simulink model "s01_unicycle"  (R2020a)
settings: Solver=VariableStepAuto  StartTime=0.0  StopTime=20  FixedStep=0.001
InitFcn:
  | clc, close all
  | 
  | run('./s00_config.m')
  | 
  | load('./parameters/ut_obj')
  | load('./parameters/yt_obj')
  | load('./parameters/Kp')
  | load('./parameters/Kr')
  | load('./parameters/Mp')
  | load('./parameters/Mr')
  | 
  | iterSeed = randi(500);
model workspace (MAT data in the model file):
  M = sym
  M.s = 'symobj::fromString("eJytkMGKwjAQhqdWxRW8KYue8gw+wS548ewDlJTMriNJCp262ptP4UP5VCZtwTTiYcGBjxkmP/NnJgWAAcDl6vIwTUYufa2gjdTV8652GvjwcM2SmX5t0+69rz0npFKJP1mSzDUKKw2yODIqQVZwbYr8sDkaU28V2op+CEsIPQfRzKFnX2gVaV79sdGzLqqoP/ZwpTTljd8UHjHzMFa72nxrkozc7rYMPG6B/m0HW3he3uR/R4m9m4UzsgrPT74TT+aMpeXMvX0GM9Jgz0R0Oep30dd2Q5I7SlFCoD==", 2)'
  M.Digits = 32
  M_nonlin = sym
  M_nonlin.s = 'symobj::fromString("eJytkMGKwjAQhqdWxRW8KYue8gw+wS548ewDlJTMriNJCp262ptP4UP5VCZtwTTiYcGBjxkmP/NnJgWAAcDl6vIwTUYufa2gjdTV8652GvjwcM2SmX5t0+69rz0npFKJP1mSzDUKKw2yODIqQVZwbYr8sDkaU28V2op+CEsIPQfRzKFnX2gVaV79sdGzLqqoP/ZwpTTljd8UHjHzMFa72nxrkozc7rYMPG6B/m0HW3he3uR/R4m9m4UzsgrPT74TT+aMpeXMvX0GM9Jgz0R0Oep30dd2Q5I7SlFCoD==", 2)'
  M_nonlin.Digits = 32
  M_tmp = sym
  M_tmp.s = 'symobj::fromString("eJytUMGKwkAMTa0uruBNcfU037BfsIIXz35AmTJxjcxMoamrvfkVfpRf5UxbcBzxIGzg8ULyyEuSAkAP4Hxx3E+TgaOfBbSRunzS5U4Dnx5cs2SmX9uUH/rfHkekUok/WZLMNQorDbI4MCpBVnBtiny/OhhTrxXairaEJYSevWhm32NXaBVpXu3Y6FkXVVT/8OBKacobvxHcY+zBWG1qs9QkGbm9bR54XAP9vz1s6vHyJ+89JfZuDs7IKjw9+Q49MmcsLWeuNwtmpMGdieg4qnfxqP3q+AZKWUKh", 2)'
  M_tmp.Digits = 32
  RHS = sym
  RHS.s = 'symobj::fromString("eJytUMGKwkAMTa2KK3hTFj3NN/gFu+DFsx9Qpkx2jcxMoamrvfkVfpRf5UxbcDriYcHAIyF55CUvBYABwOXq8jBNRi59raCN1NXzrnYc+PDgmiUz/dqm3ZuvPU5IpRJ/siSZaxRWGmRxZFSCrODaFPlhczSm3iq0Ff0QlhBqDqKdQ499oVXEeXVjw2ddVFF/7MGV0pQ3elN4xMyDsdrV5luTZOT2t2WgcQv4bzNs4fHSk/+ZEms3D2dkFZ6fdCcemROWljM3+wx2pMGfiehy1O+iz+3cSu5KYUKi", 2)'
  RHS.Digits = 32
  RHS_nonlin = sym
  RHS_nonlin.s = 'symobj::fromString("eJytUMGKwkAMTa2KK3hTFj3NN/gFu+DFsx9Qpkx2jcxMoamrvfkVfpRf5UxbcDriYcHAIyF55CUvBYABwOXq8jBNRi59raCN1NXzrnYc+PDgmiUz/dqm3ZuvPU5IpRJ/siSZaxRWGmRxZFSCrODaFPlhczSm3iq0Ff0QlhBqDqKdQ499oVXEeXVjw2ddVFF/7MGV0pQ3elN4xMyDsdrV5luTZOT2t2WgcQv4bzNs4fHSk/+ZEms3D2dkFZ6fdCcemROWljM3+wx2pMGfiehy1O+iz+3cSu5KYUKi", 2)'
  RHS_nonlin.Digits = 32
  RHS_tmp = sym
  RHS_tmp.s = 'symobj::fromString("eJytUMGKwkAMTa2KK3hTFj3NN/gFu+DFsx9Qpkx2jcxMoamrvfkVfpRf5UxbcDriYcHAIyF55CUvBYABwOXq8jBNRi59raCN1NXzrnYc+PDgmiUz/dqm3ZuvPU5IpRJ/siSZaxRWGmRxZFSCrODaFPlhczSm3iq0Ff0QlhBqDqKdQ499oVXEeXVjw2ddVFF/7MGV0pQ3elN4xMyDsdrV5luTZOT2t2WgcQv4bzNs4fHSk/+ZEms3D2dkFZ6fdCcemROWljM3+wx2pMGfiehy1O+iz+0OSe5KaUKj", 2)'
  RHS_tmp.Digits = 32
  Tp = sym
  Tp.s = 'symobj::fromString("eJytUMGKwkAMTa0uruBNkdXLfMN+wQpePPsBZcrENTIzhaau9uZX+FF+lTNtwXHEg7CBxwvJIy9JCgA9gPPFcT9NBo5+5tBG6vJJlzsNfHpwzZKZfm1Tfuh/exyRSiX+ZEky1yisNMjiwKgEWcG1KfL96mBMvVZoK9oSlhB69qKZfY9doVWkebVjo2ddVFH9w4MrpSlv/EZwj7EHY7WpzVKTZOT2tq/A4xro/+1hU4+XP3nvKbF3c3BGVuHpyXfokTljaTlzvVkwIw3uTETHUb2LR+2i4xtKcUKk", 2)'
  Tp.Digits = 32
  Tp_var = 0
  Tw = sym
  Tw.s = 'symobj::fromString("eJytUMGKwkAMTa0uruBNkRUP8w37BSt48ewHlCkT18jMFJq62ptf4Uf5Vc60BccRD8IGHi8kj7wkKQD0AM4Xx/00GTj6mUMbqcsnXe408OnBNUtm+rVN+aH/7XFEKpX4kyXJXKOw0iCLA6MSZAXXpsj3q4Mx9VqhrWhLWELo2Ytm9j12hVaR5tWOjZ51UUX1Dw+ulKa88RvBPcYejNWmNktNkpHb274Cj2ug/7eHTT1e/uS9p8TezcEZWYWnJ9+hR+aMpeXM9WbBjDS4MxEdR/UuHrWLjm9KeUKl", 2)'
  Tw.Digits = 32
  Tw_var = 0
  op_trim3 : handle (value not decoded)
  q1 = sym
  q1.s = 'symobj::fromString("eJytUFGKwkAMTa0uruCfIisIc4Y9wQr++O0BypSJa2RmCk1d7Z+n8FCeypm24Djih7CBxwvJIy9JCgA9gPPFcT9NBo5+5tBG6vJJlzsNfHpwzZKZfm1Tfuh/exyRSiX+ZEky1yisNMjiwKgEWcG1KfL96mBMvVZoK9oSlhB69qKZfY9doVWkebVjo2ddVFH9w4MrpSlv/EZwj7EHY7WpzVKTZOT2tq/A4xro/+1hU4+XP3nvKbF3c3BGVuHpyXfokTljaTlzvVkwIw3uTETHUb2LR+2i4xtKgUKm", 2)'
  q1.Digits = 32
  q1_d = sym
  q1_d.s = 'symobj::fromString("eJytUMGKwkAMTa0uruBNkfUg8w37BSt48ewHlCkT18jMFJq62ptf4Uf5Vc60BccRD8IGHi8kj7wkKQD0AM4Xx/00GTj6mUMbqcsnXe408OnBNUtm+rVN+aH/7XFEKpX4kyXJXKOw0iCLA6MSZAXXpsj3q4Mx9VqhrWhLWELo2Ytm9j12hVaR5tWOjZ51UUX1Dw+ulKa88RvBPcYejNWmNktNkpHb274Cj2ug/7eHTT1e/uS9p8TezcEZWYWnJ9+hR+aMpeXM9WbBjDS4MxEdR/UuHrWLjm9KiUKn", 2)'
  q1_d.Digits = 32
  q2 = sym
  q2.s = 'symobj::fromString("eJytUMGKwkAMTa0uruBNkfXifMN+wQpePPsBZcrENTIzhaau9uZX+FF+lTNtwXHEg7CBxwvJIy9JCgA9gPPFcT9NBo5+5tBG6vJJlzsNfHpwzZKZfm1Tfuh/exyRSiX+ZEky1yisNMjiwKgEWcG1KfL96mBMvVZoK9oSlhB69qKZfY9doVWkebVjo2ddVFH9w4MrpSlv/EZwj7EHY7WpzVKTZOT2tq/A4xro/+1hU4+XP3nvKbF3c3BGVuHpyXfokTljaTlzvVkwIw3uTETHUb2LR+2i4xtKkUKo", 2)'
  q2.Digits = 32
  q2_d = sym
  q2_d.s = 'symobj::fromString("eJytUEGOwjAMdGlBLBK3RQhOeQMvYCUunHlAlSpmMUpSqS679MYr+BO8apNSiZAVByQsjezYI088KQD0AE5nl7M06bu0nMMtUld/drXjwIcHNyyZ6du27Yf5wuMXqVLiR1YkC43CSoMsDoxKkBXcmLLYrw7GNGuFtqYtYQWhZi/amXnsSq0izrM/tnzWZR31Bx5cK01FqzeCe4w9GOtNY740SUa+3TYLNK4B/22GTTyeevKaKbF2e3BOVuHxn+7QI3fC0nLuZtNgRxrcmYguR/0ulpfgMfgDP01DUz==", 2)'
  q2_d.Digits = 32
  q3 = sym
  q3.s = 'symobj::fromString("eJytUEuKAkEMTds6zAjuFBlXNVeYEyi4ce0BmmoqjpGqaui0n955Cg/lqazqbrAscSFM4PFC8shLkgJAD+B8cdxPk4Gj+QzaSF0+7nKngS8Prlky059tyg/9X48jUqnEQZYkc43CSoMs9oxKkBVcmyLfLffG1CuFtqINYQmhZy+a2ffYFlpFmlc7NnrWRRXVPzy4Upryxm8I9xh5MFbr2iw0SUZub/sOPK6B/t8eNvF4+ZP3nhJ7NwdnZBWennw/PTJnLC1nrjcNZqTBnYnoOKp38aj96fgGSqFCqj==", 2)'
  q3.Digits = 32
  q3_d = sym
  q3_d.s = 'symobj::fromString("eJytUEuKAkEMTds6zAjuFBlXxRxhTqDgxrUHaKqpOEaqqqHTfnrnKTyUp7Kqu8GyxIUwgccLySMvSQoAPYDzxXE/TQaO5jNoI3X5uMudBr48uGbJTH+2KT/0fz2OSKUSB1mSzDUKKw2y2DMqQVZwbYp8t9wbU68U2oo2hCWEnr1oZt9jW2gVaV7t2OhZF1VU//DgSmnKG78h3GPkwVita7PQJBm5ve078LgG+n972MTj5U/ee0rs3RyckVV4evL99MicsbScud40mJEGdyai46jexaP2p+MbSqlCqz==", 2)'
  q3_d.Digits = 32
  q4 = sym
  q4.s = 'symobj::fromString("eJytUEuKAkEMTds6zAjuFBlXBXODOYGCG9ceoKmm4hipqoZO++mdp/BQnsqq7gbLEhfCBB4vJI+8JCkA9ADOF8f9NBk4ms+gjdTl4y53Gvjy4JolM/3ZpvzQ//U4IpVKHGRJMtcorDTIYs+oBFnBtSny3XJvTL1SaCvaEJYQevaimX2PbaFVpHm1Y6NnXVRR/cODK6Upb/yGcI+RB2O1rs1Ck2Tk9rbvwOMa6P/tYROPlz957ymxd3NwRlbh6cn30yNzxtJy5nrTYEYa3JmIjqN6F4/an45vSrFCrD==", 2)'
  q4.Digits = 32
  q4_d = sym
  q4_d.s = 'symobj::fromString("eJytUEuKAkEMTds6zAjuFBlXtZgTzAkU3Lj2AE01FcdIVTV02k/vPIWH8lRWdTdYlrgQJvB4IXnkJUkBoAdwvjjup8nA0XwGbaQuH3e508CXB9csmenPNuWH/q/HEalU4iBLkrlGYaVBFntGJcgKrk2R75Z7Y+qVQlvRhrCE0LMXzex7bAutIs2rHRs966KK6h8eXClNeeM3hHuMPBirdW0WmiQjt7d9Bx7XQP9vD5t4vPzJe0+JvZuDM7IKT0++nx6ZM5aWM9ebBjPS4M5EdBzVu3jU/nR8A0q5Qq0=", 2)'
  q4_d.Digits = 32
  q5 = sym
  q5.s = 'symobj::fromString("eJytUEuKAkEMTds6zAjuFBlXtZkLzAkU3Lj2AE01FcdIVTV02k/vPIWH8lRWdTdYlrgQJvB4IXnkJUkBoAdwvjjup8nA0XwGbaQuH3e508CXB9csmenPNuWH/q/HEalU4iBLkrlGYaVBFntGJcgKrk2R75Z7Y+qVQlvRhrCE0LMXzex7bAutIs2rHRs966KK6h8eXClNeeM3hHuMPBirdW0WmiQjt7d9Bx7XQP9vD5t4vPzJe0+JvZuDM7IKT0++nx6ZM5aWM9ebBjPS4M5EdBzVu3jU/nR8A0rBQq4=", 2)'
  q5.Digits = 32
  q5_d = sym
  q5_d.s = 'symobj::fromString("eJytUEuKAkEMTds6zAjuFBlXtZoDzAkU3Lj2AE01FcdIVTV02k/vPIWH8lRWdTdYlrgQJvB4IXnkJUkBoAdwvjjup8nA0XwGbaQuH3e508CXB9csmenPNuWH/q/HEalU4iBLkrlGYaVBFntGJcgKrk2R75Z7Y+qVQlvRhrCE0LMXzex7bAutIs2rHRs966KK6h8eXClNeeM3hHuMPBirdW0WmiQjt7d9Bx7XQP9vD5t4vPzJe0+JvZuDM7IKT0++nx6ZM5aWM9ebBjPS4M5EdBzVu3jU/nR8A0rJQq8=", 2)'
  q5_d.Digits = 32
  z = [0  0  0  0  0  0  0  0  0  0; 0  0  0  0  0  0  0  0  0  0; 0  0  0  0  0  0  0  0  0  0; 0  0  0  0  0  0  0  0  0  0; 0  0  0  0  0  0  0  0  0  0; 0  0  0  0  0  0  0  0  0  0; 0  0  0  0  0  0  0  0  0  0; 0  0  0  0  0  0  0  0  0  0; 0  0  0  0  0  0  0  0  0  0; 0  0  0  0  0  0  0  0  0  0]
values from neighbouring files (symbols this model uses):
  b_disc = 0.01    [s00_config.m]
  Bp = [B_p1 B_p2 B_p3 B_p4]    [s00_config.m]    (also in s00_designLQR.m = double([0; b2; 0; b4]))
  flag_AddPitchBias = 0    [s00_config.m]
  flag_AddRollBias = 0    [s00_config.m]
  flag_UseAccNoise = 1    [s00_config.m]
  flag_useControlDelay = 0    [s00_config.m]
  flag_UseGyroNoise = 1    [s00_config.m]
  flag_UsePitchEst = 1    [s00_config.m]
  flag_UsePivotAcc = 1    [s00_config.m]
  flag_UseRateEst = 1    [s00_config.m]
  flag_UseRollEst = 1    [s00_config.m]
  flag_UseYawEst = 1    [s00_config.m]
  Icx = 0.001746    [s00_config.m]
  Icy = 0.00181    [s00_config.m]
  Icz = 0.001585    [s00_config.m]
  Iwx = 0.000259    [s00_config.m]
  Iwy = 0.000503    [s00_config.m]
  Iwz = 0.000259    [s00_config.m]
  Lc = 0.055    [s00_config.m]
  Lcp = 0.055    [s00_config.m]
  mean_IMUgyro = -0.0065    [s00_config.m]
  pitch_bias = deg2rad(1)    [s00_config.m]
  q1_0 = -deg2rad(36)    [s00_config.m]
  q2_0 = deg2rad(0)    [s00_config.m]
  r = Rw - 0.01    (= 0.043)    [s00_config.m]
  roll_bias = deg2rad(1)    [s00_config.m]
  Rw = 0.053    [s00_config.m]
  stall_torque = 1.6    [s00_config.m]
  Ts = 1/100    (= 0.01)    [s00_config.m]
  variance_IMUacc = 0.0049    [s00_config.m]
  variance_IMUgyro = 6.3956e-04    (= 0.00063956)    [s00_config.m]
  X = (P.')/(P*P.')    [s00_config.m]
  Xp = X(:,1)    [s00_config.m]
undefined symbols (not defined in the file or in its folder): DiscIntNeverNeededParam, sigbuilder_block, Y, Z
libraries: sm_lib x59, aerolibconvert2 x11, nesl_utility x8, eeGeneralControl x2, simulink x1, SignalEditorBlockLib x1
(part 1 of 2)
settings Model: Creator=zjia  LastModifiedBy=Geist
settings DataIOCC: ExternalInput=getinputstruct(op_trim3)  InitialState=getstatestruct(op_trim3)  ReturnWorkspaceOutputs=off
settings DebuggingCC: PregeneratedLibrarySubsystemCodeDiagnostic=none  ArithmeticOperatorsInVariantConditions=warning
settings SFSimCC: SimUseLocalCustomCode=off  CustomCodeUndefinedFunction=UseInterfaceOnly
settings RTWCC: RTWUseLocalCustomCode=off
settings ExplorerConfigSet: InternalSimMechanicsExplorerSettings="<ExplorerConfiguration><canonicalview>default</canonicalview><AnimationSetting><BasePlaybackSpeed>1.0</BasePlaybackSpeed><PlaybackSpeedFactor>1.0</PlaybackSpeedFactor></AnimationSetting><TilePanel><TileInfo><Tiles Columns=\"1\" Count=\"1\" Rows=\"1\"><Column Weight=\"1\"/><Row Weight=\"1\"/><Tile Height=\"1\" Width=\"1\" X=\"0\" Y=\"0\"/></Tiles></TileInfo><SceneInfo><SceneViewer><BGColor><R>0.60000002384185791</R><G>0.60000002384185791</G><B>0.60000002384185791</B></BGColor><Camera><DoPerspective>off</DoPerspective><Position><X>-1.31570593920536782</X><Y>-1.95913294447027075</Y><Z>2.91484294326524562</Z></Position><Center><X>-0.265965718532476025</X><Y>-0.0141378650214136238</Y><Z>0.259288232843852717</Z></Center><Up><X>0.409238570116308875</X><Y>0.651418880522143251</Y><Z>0.638887497786924219</Z></Up><ViewLimDist>1</ViewLimDist><YLim>0.274439838409632098</YLim><XLim>0.321907563939727526</XLim></Camera></SceneViewer></SceneInfo></TilePanel><MechEditorPanel><Cameras/><GfxPanelCameraMap/><VideoCreator><PlaybackSpeedRatio>1.0</PlaybackSpeedRatio><FrameRate>30</FrameRate><VideoFormat>Motion JPEG AVI</VideoFormat><FrameSize>auto</FrameSize></VideoCreator></MechEditorPanel></ExplorerConfiguration>"

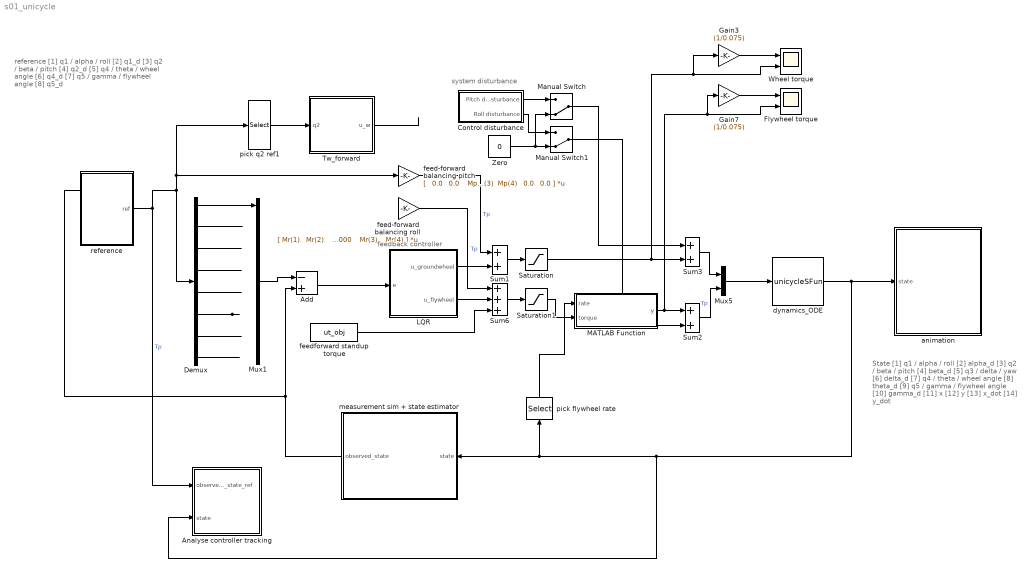
== system s01_unicycle ==
  note: State
      |
      | [1] q1 / alpha / roll
      | [2] alpha_d
      | [3] q2 / beta / pitch
      | [4] beta_d
      | [5] q3 / delta / yaw
      | [6] delta_d
      | [7] q4 / theta / wheel angle
      | [8] theta_d
      | [9] q5 / gamma / flywheel angle
      | [10] gamma_d
      | [11] x
      | [12] y
      | [13] x_dot
      | [14] y_dot
  note: feedback controller
  note: reference
      |
      | [1] q1 / alpha / roll
      | [2] q1_d
      | [3] q2 / beta / pitch
      | [4] q2_d
      | [5] q4 / theta / wheel angle
      | [6] q4_d
      | [7] q5 / gamma / flywheel angle
      | [8] q5_d
  note: system disturbance
  Add : Sum  Inputs=-+
  Analyse controller tracking : Subsystem
  Control disturbance : Subsystem  Tag=STV Subsys  LoadFcn=sigbuilder_block('load');  StartFcn=sigbuilder_block('start');  StopFcn=sigbuilder_block('stop');  ClipboardFcn=sigbuilder_block('clipboard');  mask(Sigbuilder block){tuvar=[0:10]}
      mask help: Simulink:masks:SigbuilderBlock_MD
      mask init:
      | if ~strcmp(get_param(bdroot(gcbh),'SimulationStatus'),'stopped') tuvar = sigbuilder_block('maskInit'); end
      settings: CopyFcn=sigbuilder_block('copy');  DeleteFcn=sigbuilder_block('delete');  ModelCloseFcn=sigbuilder_block('modelClose');  PreSaveFcn=sigbuilder_block('preSave');  PauseFcn=sigbuilder_block('pause');  ContinueFcn=sigbuilder_block('continue');  NameChangeFcn=sigbuilder_block('namechange');  OpenFcn=sigbuilder_block('open',[437.6 199.2 550.4 400 ]);  CloseFcn=sigbuilder_block('close');
      mask Display: plot(0, 0, 100, 100,[2, 2, 32, 32, 2], [68, 8, 8, 68, 68],[32, 2], [38, 38], [32, 19, 2],[53, 60, 44], [32, 17, 17, 2],[16, 16, 31, 31]);txt = getActiveGroup(gcbh);text(2, 100, txt,'verticalAlignment', 'top');
  Demux : Demux  Outputs=8
  Flywheel torque : Scope  NumInputPorts=2
  Gain3 : Gain  Gain=(1/0.075)
  Gain7 : Gain  Gain=(1/0.075)
  LQR : Subsystem
  MATLAB Function : MATLAB Function  TreatAsAtomicUnit=on
  Manual Switch : ManualSwitch  CurrentSetting=0
  Manual Switch1 : ManualSwitch  CurrentSetting=0
  Mux1 : Mux  Inputs=8
  Mux5 : Mux  Inputs=2
  Saturation : Saturate  UpperLimit=stall_torque  LowerLimit=-stall_torque
  Saturation1 : Saturate  UpperLimit=stall_torque  LowerLimit=-stall_torque
  Sum1 : Sum
  Sum2 : Sum
  Sum3 : Sum
  Sum6 : Sum  Inputs=+++
  Tw_forward : MATLAB Function  TreatAsAtomicUnit=on
  Wheel torque : Scope  NumInputPorts=2
  Zero : Constant  Value=0  OutDataTypeStr=Inherit: Inherit via back propagation
  animation : Subsystem
      mask Display: image('C:\Users\geist\Documents\code_projects\uniwheel_model\simulink_3D_unicycle\images\simulation_block_image.PNG'); % Use "Edit Image" on toolstrip to change.
  dynamics_ODE : S-Function  FunctionName=unicycleSFun  SFunctionDeploymentMode=off  EnableBusSupport=off
  feed-forward balancing pitch : Gain  Gain=|  Multiplication=Matrix(K*u) (u vector)
      | [   0.0   0.0    Mp(1)   Mp(2)   Mp(3)  Mp(4)   0.0   0.0
      | ]
  feed-forward balancing roll : Gain  Gain=|  Multiplication=Matrix(K*u) (u vector)
      | [ Mr(1)   Mr(2)    0.0000    0.0000    0.0000    0.0000    Mr(3)    Mr(4)
      | ]
  feedforward standup torque : FromWorkspace  VariableName=ut_obj
  measurement sim + state estimator : Subsystem
  pick flywheel rate : Selector  InputPortWidth=14  IndexOptions=Index vector (dialog)  Indices=[10]  OutputSizes=1
  pick q2 ref1 : Selector  InputPortWidth=8  IndexOptions=Index vector (dialog)  Indices=[3]  OutputSizes=1
  reference : Subsystem
  wires:
  Mux5/1 -> dynamics_ODE/1
  Sum3/1 -> Mux5/1
  measurement sim + state estimator/1(observed_state) -> Add/2
  Sum2/1 -> Mux5/2  "Tp"
  Manual Switch1/1 -> Sum2/2
  MATLAB Function/1(y) -> Sum2/1, Flywheel torque/2, Gain7/1
  Control disturbance/1(Pitch disturbance) -> Manual Switch/1
  Manual Switch/1 -> Sum3/1
  Zero/1 -> Manual Switch1/2, Manual Switch/2
  Control disturbance/2(Roll disturbance) -> Manual Switch1/1
  Gain3/1 -> Wheel torque/1
  Gain7/1 -> Flywheel torque/1
  pick flywheel rate/1 -> MATLAB Function/1(rate)
  feedforward standup torque/1 -> Sum6/3
  Sum6/1 -> Saturation1/1
  Add/1 -> LQR/1(e)
  feed-forward balancing pitch/1 -> Sum1/1  "Tp"
  Sum1/1 -> Saturation/1
  feed-forward balancing roll/1 -> Sum6/1  "Tp"
  dynamics_ODE/1 -> Analyse controller tracking/2(state), pick flywheel rate/1, measurement sim + state estimator/1(state), animation/1(state)
  LQR/1(u_groundwheel) -> Sum1/2
  LQR/2(u_flywheel) -> Sum6/2
  Saturation/1 -> Sum3/2, Gain3/1, Wheel torque/2
  Saturation1/1 -> MATLAB Function/2(torque)
  reference/1(ref) -> feed-forward balancing pitch/1, pick q2 ref1/1, Demux/1, Analyse controller tracking/1(observed_state_ref)  "Tp"
  Demux/3 -> ?
  Demux/6 -> ?
  Mux1/1 -> Add/1
  Demux/2 -> ?
  Demux/1 -> Mux1/1
  Demux/8 -> ?
  Demux/7 -> ?
  Demux/5 -> ?
  Demux/4 -> ?
  Tw_forward/1(u_w) -> ?
  pick q2 ref1/1 -> Tw_forward/1(q2)

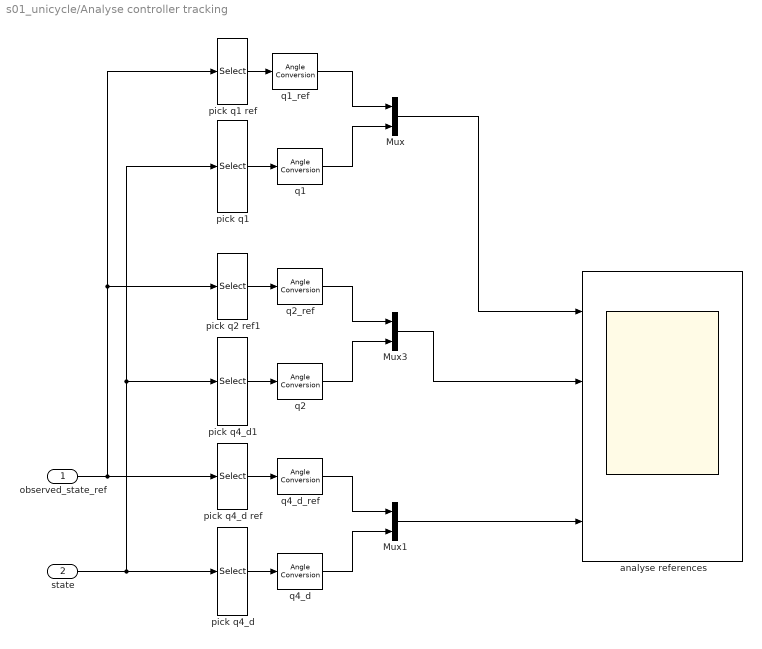
== system s01_unicycle/Analyse controller tracking ==
  observed_state_ref : Inport
  state : Inport  Port=2
  Mux : Mux  Inputs=2
  Mux1 : Mux  Inputs=2
  Mux3 : Mux  Inputs=2
  analyse references : Scope  NumInputPorts=4
  pick q1 : Selector  InputPortWidth=14  IndexOptions=Index vector (dialog)  Indices=[1]  OutputSizes=1
  pick q1 ref : Selector  InputPortWidth=8  IndexOptions=Index vector (dialog)  Indices=[1]  OutputSizes=1
  pick q2 ref1 : Selector  InputPortWidth=8  IndexOptions=Index vector (dialog)  Indices=[3]  OutputSizes=1
  pick q4_d : Selector  InputPortWidth=14  IndexOptions=Index vector (dialog)  Indices=[8]  OutputSizes=1
  pick q4_d ref : Selector  InputPortWidth=8  IndexOptions=Index vector (dialog)  Indices=[6]  OutputSizes=1
  pick q4_d1 : Selector  InputPortWidth=14  IndexOptions=Index vector (dialog)  Indices=[3]  OutputSizes=1
  q1 : aerolibconvert2/Angle Conversion  IU=rad  OU=deg
  q1_ref : aerolibconvert2/Angle Conversion  IU=rad  OU=deg
  q2 : aerolibconvert2/Angle Conversion  IU=rad  OU=deg
  q2_ref : aerolibconvert2/Angle Conversion  IU=rad  OU=deg
  q4_d : aerolibconvert2/Angle Conversion  IU=rad  OU=deg
  q4_d_ref : aerolibconvert2/Angle Conversion  IU=rad  OU=deg
  wires:
  pick q4_d ref/1 -> q4_d_ref/1
  pick q4_d/1 -> q4_d/1
  q1/1 -> Mux/2
  pick q1/1 -> q1/1
  observed_state_ref/1 -> pick q2 ref1/1, pick q1 ref/1, pick q4_d ref/1
  pick q1 ref/1 -> q1_ref/1
  q4_d_ref/1 -> Mux1/1
  q1_ref/1 -> Mux/1
  q4_d/1 -> Mux1/2
  Mux1/1 -> analyse references/4
  Mux/1 -> analyse references/1
  Mux3/1 -> analyse references/2
  q2/1 -> Mux3/2
  q2_ref/1 -> Mux3/1
  state/1 -> pick q4_d1/1, pick q1/1, pick q4_d/1
  pick q4_d1/1 -> q2/1
  pick q2 ref1/1 -> q2_ref/1

== system s01_unicycle/Control disturbance ==
  Demux : Demux  Tag=STV Demux  Outputs=2
      settings: DisplayOption=none
  FromWs : FromWorkspace  Tag=STV FromWs  VariableName=tuvar
      SigBuilderData=|
      | common.afterFinalStr = 'Extrapolate'
      | common.sampleTime = 0
      | dataSet.timeRange = [0 10]
      | dataSet.name = 'Group 1'
      | sbobj.Groups.Name = 'Group 1'
      | sbobj.Groups.Signals(1).Name = 'Pitch disturbance'
      | sbobj.Groups.Signals(1).XData = [0 2.9 3 3.1 3.2 10]
      | sbobj.Groups.Signals(1).YData = [0 0 0.272 0.128 0 0]
      | sbobj.Groups.Signals(2).Name = 'Roll disturbance'
      | sbobj.Groups.Signals(2).XData = [0 2.9 3 3.2 3.3 10]
      | sbobj.Groups.Signals(2).YData = [0 0 0.505 0.185 0 0]
  Pitch disturbance : Outport  Tag=STV Outport
  Roll disturbance : Outport  Tag=STV Outport  Port=2
  wires:
  Demux/1 -> Pitch disturbance/1
  FromWs/1 -> Demux/1
  Demux/2 -> Roll disturbance/1

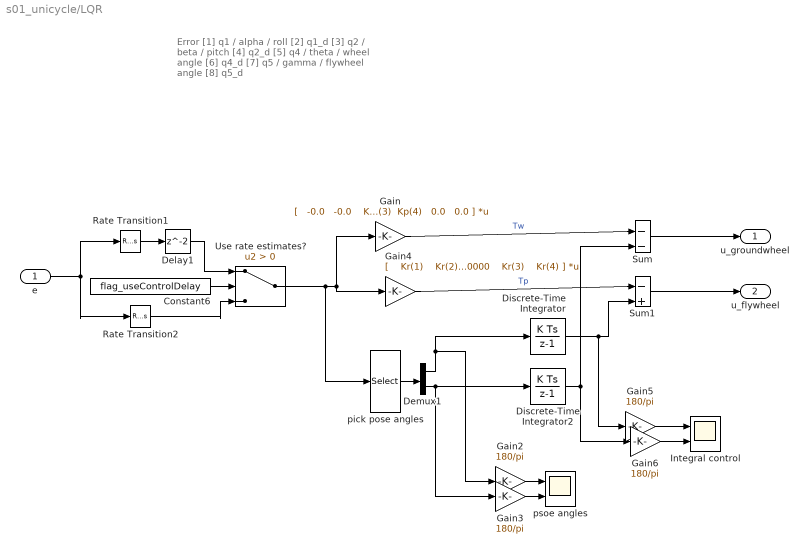
== system s01_unicycle/LQR ==
  note: Error
      |
      | [1] q1 / alpha / roll
      | [2] q1_d
      | [3] q2 / beta / pitch
      | [4] q2_d
      | [5] q4 / theta / wheel angle
      | [6] q4_d
      | [7] q5 / gamma / flywheel angle
      | [8] q5_d
  e : Inport
  Constant6 : Constant  Value=flag_useControlDelay
  Delay1 : Delay  SampleTime=Ts
  Demux1 : Demux  Outputs=2
  Discrete-Time Integrator : DiscreteIntegrator  gainval=gain_int_roll  SampleTime=-1  ICPrevOutput=DiscIntNeverNeededParam  ICPrevScaledInput=DiscIntNeverNeededParam
  Discrete-Time Integrator2 : DiscreteIntegrator  gainval=gain_int_pitch  SampleTime=-1  ICPrevOutput=DiscIntNeverNeededParam  ICPrevScaledInput=DiscIntNeverNeededParam
  Gain : Gain  Gain=|  Multiplication=Matrix(K*u) (u vector)
      | [   -0.0   -0.0    Kp(1)   Kp(2)   Kp(3)  Kp(4)   0.0   0.0
      | ]
  Gain{2..3,5..6} (4 alike) : Gain  Gain=180/pi
  Gain4 : Gain  Gain=|  Multiplication=Matrix(K*u) (u vector)
      | [    Kr(1)    Kr(2)    0.0000    0.0000    0.0000    0.0000    Kr(3)    Kr(4)
      | ]
  Integral control : Scope  NumInputPorts=2
  Rate Transition1 : RateTransition  OutPortSampleTime=Ts
  Rate Transition2 : RateTransition  OutPortSampleTime=Ts
  Sum : Sum  Inputs=|--
  Sum1 : Sum  Inputs=|-+
  Use rate estimates? : Switch  Criteria=u2 > Threshold
  pick pose angles : Selector  InputPortWidth=8  IndexOptions=Index vector (dialog)  Indices=[1,3]  OutputSizes=1
  psoe angles : Scope  NumInputPorts=2
  u_groundwheel : Outport  VectorParamsAs1DForOutWhenUnconnected=off
  u_flywheel : Outport  Port=2  VectorParamsAs1DForOutWhenUnconnected=off
  wires:
  e/1 -> Rate Transition2/1, Rate Transition1/1
  Gain4/1 -> Sum1/1  "Tp"
  Delay1/1 -> Use rate estimates?/1
  Gain/1 -> Sum/1  "Tw"
  Rate Transition1/1 -> Delay1/1
  Constant6/1 -> Use rate estimates?/2
  Rate Transition2/1 -> Use rate estimates?/3
  pick pose angles/1 -> Demux1/1
  Discrete-Time Integrator/1 -> Sum1/2, Gain5/1
  Demux1/1 -> Gain2/1, Discrete-Time Integrator/1
  Demux1/2 -> Gain3/1, Discrete-Time Integrator2/1
  Discrete-Time Integrator2/1 -> Gain6/1, Sum/2
  Use rate estimates?/1 -> pick pose angles/1, Gain4/1, Gain/1
  Gain2/1 -> psoe angles/1
  Gain3/1 -> psoe angles/2
  Gain5/1 -> Integral control/1
  Gain6/1 -> Integral control/2
  Sum1/1 -> u_flywheel/1
  Sum/1 -> u_groundwheel/1

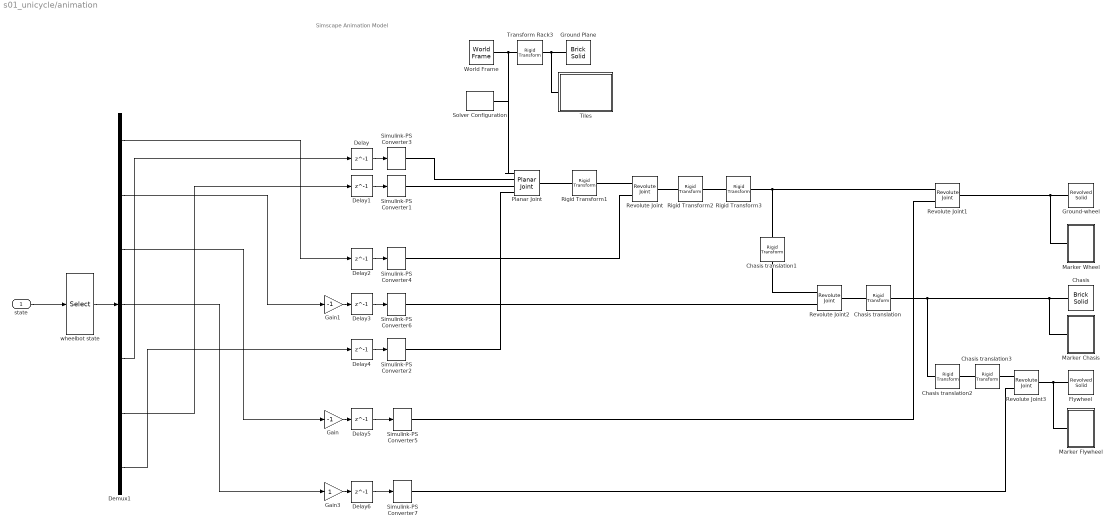
== system s01_unicycle/animation ==
  note: Simscape Animation Model
  state : Inport
  Chasis : sm_lib/Body Elements/Brick Solid  GraphicAmbientColor=[0.15 0.15 0.15 1.0]  BasedOnType=Density  BrickDimensions=[0.04 Lcp+Lc 0.04]  BrickDimensionUnits=m  CenterOfMass=[0 (Lcp-Lc)/2 0]  CenterOfMassUnits=m  GraphicDiffuseColor=[0.0 0.8 0.2]  Density=0  DensityUnits=kg/(m^3)  DoExposeReferenceFrame=on  GraphicEmissiveColor=[0.0 0.0 0.0 1.0]  ExportEntireGeometry=off  SerializedFrames=<Frames/>  MarkerShape=Sphere  MarkerSize=10  GraphicType=FromGeometry  InertiaType=PointMass  Mass=0  MassUnits=kg  MomentsOfInertia=[Icx Icz Icy]  MomentsOfInertiaUnits=kg*m^2  GraphicOpacity=1.0  ProductsOfInertia=[0 0 0]  ProductsOfInertiaUnits=kg*m^2  GraphicShininess=75  GraphicSpecularColor=[0.5 0.5 0.5 1.0]  GraphicVisPropType=SimpleVisualProperties
  Chasis translation : sm_lib/Frames and Transforms/Rigid Transform  TranslationMethod=StandardAxis  TranslationStandardOffset=(Lcp+Lc)/2  TranslationLengthUnit=m  TranslationStandardAxis=+Y  TranslationCartesianOffset=[0 0 0]  TranslationROffset=0  TranslationROffsetUnits=m  TranslationZOffset=0  TranslationZOffsetUnits=m  TranslationThetaOffset=0  TranslationThetaOffsetUnits=deg  RotationMethod=None  RotationAngleUnits=deg  RotationStandardAxis=+Z  RotationAngle=0  RotationArbitraryAxis=[0 0 1]  FollAlignAxisA=+X  BaseAlignAxisA=+Y  FollAlignAxisB=+Y  BaseAlignAxisB=+Z  RotationSequenceAxes=FollowerAxes  RotationSequence=XYX  RotationSequenceAngles=[0 0 0]  RotationSequenceAnglesUnits=deg  RotationMatrix=[1 0 0; 0 1 0; 0 0 1]
  Chasis translation1 : sm_lib/Frames and Transforms/Rigid Transform  TranslationMethod=None  TranslationStandardOffset=(Lcp+Lc)/2  TranslationLengthUnit=m  TranslationStandardAxis=+Y  TranslationCartesianOffset=[0 0 0]  TranslationROffset=0  TranslationROffsetUnits=m  TranslationZOffset=0  TranslationZOffsetUnits=m  TranslationThetaOffset=0  TranslationThetaOffsetUnits=deg  RotationMethod=StandardAxis  RotationAngleUnits=deg  RotationStandardAxis=+Z  RotationAngle=90  RotationArbitraryAxis=[0 0 1]  FollAlignAxisA=+X  BaseAlignAxisA=+Y  FollAlignAxisB=+Y  BaseAlignAxisB=+Z  RotationSequenceAxes=FollowerAxes  RotationSequence=XYX  RotationSequenceAngles=[0 0 0]  RotationSequenceAnglesUnits=deg  RotationMatrix=[1 0 0; 0 1 0; 0 0 1]
  Chasis translation2 : sm_lib/Frames and Transforms/Rigid Transform  TranslationMethod=StandardAxis  TranslationStandardOffset=(Lcp+Lc)/2  TranslationLengthUnit=m  TranslationStandardAxis=+Y  TranslationCartesianOffset=[0 0 0]  TranslationROffset=0  TranslationROffsetUnits=m  TranslationZOffset=0  TranslationZOffsetUnits=m  TranslationThetaOffset=0  TranslationThetaOffsetUnits=deg  RotationMethod=None  RotationAngleUnits=deg  RotationStandardAxis=+Z  RotationAngle=0  RotationArbitraryAxis=[0 0 1]  FollAlignAxisA=+X  BaseAlignAxisA=+Y  FollAlignAxisB=+Y  BaseAlignAxisB=+Z  RotationSequenceAxes=FollowerAxes  RotationSequence=XYX  RotationSequenceAngles=[0 0 0]  RotationSequenceAnglesUnits=deg  RotationMatrix=[1 0 0; 0 1 0; 0 0 1]
  Chasis translation3 : sm_lib/Frames and Transforms/Rigid Transform  TranslationMethod=None  TranslationStandardOffset=(Lcp+Lc)/2  TranslationLengthUnit=m  TranslationStandardAxis=+Y  TranslationCartesianOffset=[0 0 0]  TranslationROffset=0  TranslationROffsetUnits=m  TranslationZOffset=0  TranslationZOffsetUnits=m  TranslationThetaOffset=0  TranslationThetaOffsetUnits=deg  RotationMethod=StandardAxis  RotationAngleUnits=deg  RotationStandardAxis=+Y  RotationAngle=90  RotationArbitraryAxis=[0 0 1]  FollAlignAxisA=+X  BaseAlignAxisA=+Y  FollAlignAxisB=+Y  BaseAlignAxisB=+Z  RotationSequenceAxes=FollowerAxes  RotationSequence=XYX  RotationSequenceAngles=[0 0 0]  RotationSequenceAnglesUnits=deg  RotationMatrix=[1 0 0; 0 1 0; 0 0 1]
  Delay{,1..6} (7 alike) : Delay  DelayLength=1
  Demux1 : Demux  Outputs=7
  Flywheel : sm_lib/Body Elements/Revolved Solid  GraphicAmbientColor=[0.15 0.15 0.15 1.0]  BasedOnType=Density  CenterOfMass=[0 0 0]  CenterOfMassUnits=m  GraphicDiffuseColor=[1.0 0.0 0.0]  ExportConvexHullGeometry=off  Density=1000  DensityUnits=kg/(m^3)  DoExposeReferenceFrame=on  GraphicEmissiveColor=[0.0 0.0 0.0 1.0]  ExportEntireGeometry=off  SerializedFrames=<Frames/>  MarkerShape=Frame  MarkerSize=10  GraphicType=FromGeometry  InertiaType=PointMass  Mass=0  MassUnits=kg  MomentsOfInertia=[Iwx Iwz Iwy]  MomentsOfInertiaUnits=kg*m^2  GraphicOpacity=1.0  ProductsOfInertia=[0 0 0]  ProductsOfInertiaUnits=kg*m^2  RevolutionCrossSection=[r b_disc/2; r -b_disc/2; Rw -b_disc/2; Rw b_disc/2]  RevolutionCrossSectionUnits=m  RevolutionAngle=180  RevolutionAngleUnits=deg  RevolutionExtent=Full  GraphicShininess=75  GraphicSpecularColor=[0.5 0.5 0.5 1.0]  GraphicVisPropType=SimpleVisualProperties
  Gain : Gain  Gain=-1
  Gain1 : Gain  Gain=-1
  Gain3 : Gain
  Ground Plane : sm_lib/Body Elements/Brick Solid  GraphicAmbientColor=[0.15 0.15 0.15 1.0]  BasedOnType=Density  BrickDimensions=[5 5 0.001]  BrickDimensionUnits=m  CenterOfMass=[0 0 0]  CenterOfMassUnits=m  GraphicDiffuseColor=[0.8 0.8 0.8]  Density=100  DensityUnits=kg/(m^3)  DoExposeReferenceFrame=on  GraphicEmissiveColor=[0.0 0.0 0.0 1.0]  ExportEntireGeometry=off  SerializedFrames=<Frames/>  MarkerShape=Cube  MarkerSize=10000  GraphicType=FromGeometry  InertiaType=CalculateFromGeometry  Mass=1  MassUnits=kg  MomentsOfInertia=[1 1 1]  MomentsOfInertiaUnits=kg*m^2  GraphicOpacity=1  ProductsOfInertia=[0 0 0]  ProductsOfInertiaUnits=kg*m^2  GraphicShininess=75  GraphicSpecularColor=[0.5 0.5 0.5 1.0]  GraphicVisPropType=SimpleVisualProperties
  Ground-wheel : sm_lib/Body Elements/Revolved Solid  GraphicAmbientColor=[0.15 0.15 0.15 1.0]  BasedOnType=Density  CenterOfMass=[0 0 0]  CenterOfMassUnits=m  GraphicDiffuseColor=[0.0 0.4 1.0]  ExportConvexHullGeometry=off  Density=1000  DensityUnits=kg/(m^3)  DoExposeReferenceFrame=on  GraphicEmissiveColor=[0.0 0.0 0.0 1.0]  ExportEntireGeometry=off  SerializedFrames=<Frames/>  MarkerShape=Frame  MarkerSize=10  GraphicType=FromGeometry  InertiaType=PointMass  Mass=0  MassUnits=kg  MomentsOfInertia=[Iwx Iwz Iwy]  MomentsOfInertiaUnits=kg*m^2  GraphicOpacity=1.0  ProductsOfInertia=[0 0 0]  ProductsOfInertiaUnits=kg*m^2  RevolutionCrossSection=[r b_disc/2; r -b_disc/2; Rw -b_disc/2; Rw b_disc/2]  RevolutionCrossSectionUnits=m  RevolutionAngle=180  RevolutionAngleUnits=deg  RevolutionExtent=Full  GraphicShininess=75  GraphicSpecularColor=[0.5 0.5 0.5 1.0]  GraphicVisPropType=SimpleVisualProperties
  Marker Chasis : Subsystem
  Marker Flywheel : Subsystem
  Marker Wheel : Subsystem
  Planar Joint : sm_lib/Joints/Planar Joint  JointMode=Normal  SenseConstraintForce=off  SenseConstraintForceX=off  SenseConstraintForceY=off  SenseConstraintForceZ=off  SenseConstraintTorque=off  SenseConstraintTorqueX=off  SenseConstraintTorqueY=off  SenseConstraintTorqueZ=off  SenseTotalForce=off  SenseTotalForceX=off  SenseTotalForceY=off  SenseTotalForceZ=off  SenseTotalTorque=off  SenseTotalTorqueX=off  SenseTotalTorqueY=off  SenseTotalTorqueZ=off  CompositeWrenchDir=FollowerOnBase  CompositeWrenchFrame=BaseFrame  PxEquilibriumPosition=0  PxEquilibriumPositionUnits=m  PxSpringStiffness=0  PxSpringStiffnessUnits=N/m  PxDampingCoefficient=0  PxDampingCoefficientUnits=N/(m/s)  PxTorqueActuationMode=ComputedTorque  PxMotionActuationMode=InputMotion  PxSensePosition=off  PxSenseVelocity=off  PxSenseAcceleration=off  PxSenseTorqueForce=off  PxSenseLowerLimitTorqueForce=off  PxSenseUpperLimitTorqueForce=off  PxLowerLimitSpecify=off  PxLowerLimitBound=-1  PxLowerLimitBoundUnits=m  PxLowerLimitStiffness=1e6  PxLowerLimitStiffnessUnits=N/m  PxLowerLimitDamping=1e3  PxLowerLimitDampingUnits=N/(m/s)  PxLowerLimitTransitionRegionWidth=1e-4  PxLowerLimitTransitionRegionWidthUnits=m  PxUpperLimitSpecify=off  PxUpperLimitBound=1  PxUpperLimitBoundUnits=m  PxUpperLimitStiffness=1e6  PxUpperLimitStiffnessUnits=N/m  PxUpperLimitDamping=1e3  PxUpperLimitDampingUnits=N/(m/s)  PxUpperLimitTransitionRegionWidth=1e-4  PxUpperLimitTransitionRegionWidthUnits=m  PxPositionTargetSpecify=off  PxPositionTargetPriority=High  PxPositionTargetValue=0  PxPositionTargetValueUnits=m  PxVelocityTargetSpecify=off  PxVelocityTargetPriority=High  PxVelocityTargetValue=0  PxVelocityTargetValueUnits=m/s  PyEquilibriumPosition=0  PyEquilibriumPositionUnits=m  PySpringStiffness=0  PySpringStiffnessUnits=N/m  PyDampingCoefficient=0  PyDampingCoefficientUnits=N/(m/s)  PyTorqueActuationMode=ComputedTorque  PyMotionActuationMode=InputMotion  PySensePosition=off  PySenseVelocity=off  PySenseAcceleration=off  PySenseTorqueForce=off  PySenseLowerLimitTorqueForce=off  PySenseUpperLimitTorqueForce=off  PyLowerLimitSpecify=off  PyLowerLimitBound=-1  PyLowerLimitBoundUnits=m  PyLowerLimitStiffness=1e6  PyLowerLimitStiffnessUnits=N/m  PyLowerLimitDamping=1e3  PyLowerLimitDampingUnits=N/(m/s)  PyLowerLimitTransitionRegionWidth=1e-4  PyLowerLimitTransitionRegionWidthUnits=m  PyUpperLimitSpecify=off  PyUpperLimitBound=1  PyUpperLimitBoundUnits=m  PyUpperLimitStiffness=1e6  PyUpperLimitStiffnessUnits=N/m  PyUpperLimitDamping=1e3  PyUpperLimitDampingUnits=N/(m/s)  PyUpperLimitTransitionRegionWidth=1e-4  PyUpperLimitTransitionRegionWidthUnits=m  PyPositionTargetSpecify=off  PyPositionTargetPriority=High  PyPositionTargetValue=0  PyPositionTargetValueUnits=m  PyVelocityTargetSpecify=off  PyVelocityTargetPriority=High  PyVelocityTargetValue=0  PyVelocityTargetValueUnits=m/s  RzEquilibriumPosition=0  RzEquilibriumPositionUnits=deg  RzSpringStiffness=0  RzSpringStiffnessUnits=N*m/deg  RzDampingCoefficient=0  RzDampingCoefficientUnits=N*m/(deg/s)  RzTorqueActuationMode=ComputedTorque  RzMotionActuationMode=InputMotion  RzSensePosition=off  RzSenseVelocity=off  RzSenseAcceleration=off  RzSenseTorqueForce=off  RzSenseLowerLimitTorqueForce=off  RzSenseUpperLimitTorqueForce=off  RzLowerLimitSpecify=off  RzLowerLimitBound=-90  RzLowerLimitBoundUnits=deg  RzLowerLimitStiffness=1e4  RzLowerLimitStiffnessUnits=N*m/deg  RzLowerLimitDamping=10  RzLowerLimitDampingUnits=N*m/(deg/s)  RzLowerLimitTransitionRegionWidth=0.1  RzLowerLimitTransitionRegionWidthUnits=deg  RzUpperLimitSpecify=off  RzUpperLimitBound=90  RzUpperLimitBoundUnits=deg  RzUpperLimitStiffness=1e4  RzUpperLimitStiffnessUnits=N*m/deg  RzUpperLimitDamping=10  RzUpperLimitDampingUnits=N*m/(deg/s)  RzUpperLimitTransitionRegionWidth=0.1  RzUpperLimitTransitionRegionWidthUnits=deg  RzPositionTargetSpecify=off  RzPositionTargetPriority=High  RzPositionTargetValue=0  RzPositionTargetValueUnits=deg  RzVelocityTargetSpecify=off  RzVelocityTargetPriority=High  RzVelocityTargetValue=0  RzVelocityTargetValueUnits=deg/s
  Revolute Joint{,1..3} (4 alike) : sm_lib/Joints/Revolute Joint  JointMode=Normal  SenseConstraintForce=off  SenseConstraintForceX=off  SenseConstraintForceY=off  SenseConstraintForceZ=off  SenseConstraintTorque=off  SenseConstraintTorqueX=off  SenseConstraintTorqueY=off  SenseConstraintTorqueZ=off  SenseTotalForce=off  SenseTotalForceX=off  SenseTotalForceY=off  SenseTotalForceZ=off  SenseTotalTorque=off  SenseTotalTorqueX=off  SenseTotalTorqueY=off  SenseTotalTorqueZ=off  CompositeWrenchDir=FollowerOnBase  CompositeWrenchFrame=BaseFrame  EquilibriumPosition=0  EquilibriumPositionUnits=deg  SpringStiffness=0  SpringStiffnessUnits=N*m/deg  DampingCoefficient=0  DampingCoefficientUnits=N*m/(deg/s)  TorqueActuationMode=ComputedTorque  MotionActuationMode=InputMotion  SensePosition=off  SenseVelocity=off  SenseAcceleration=off  SenseTorqueForce=off  SenseLowerLimitTorqueForce=off  SenseUpperLimitTorqueForce=off  LowerLimitSpecify=off  LowerLimitBound=-90  LowerLimitBoundUnits=deg  LowerLimitStiffness=1e4  LowerLimitStiffnessUnits=N*m/deg  LowerLimitDamping=10  LowerLimitDampingUnits=N*m/(deg/s)  LowerLimitTransitionRegionWidth=0.1  LowerLimitTransitionRegionWidthUnits=deg  UpperLimitSpecify=off  UpperLimitBound=90  UpperLimitBoundUnits=deg  UpperLimitStiffness=1e4  UpperLimitStiffnessUnits=N*m/deg  UpperLimitDamping=10  UpperLimitDampingUnits=N*m/(deg/s)  UpperLimitTransitionRegionWidth=0.1  UpperLimitTransitionRegionWidthUnits=deg  PositionTargetSpecify=off  PositionTargetPriority=High  PositionTargetValue=0  PositionTargetValueUnits=deg  VelocityTargetSpecify=off  VelocityTargetPriority=High  VelocityTargetValue=0  VelocityTargetValueUnits=deg/s
  Rigid Transform1 : sm_lib/Frames and Transforms/Rigid Transform  TranslationMethod=None  TranslationStandardOffset=0  TranslationLengthUnit=m  TranslationStandardAxis=+Z  TranslationCartesianOffset=[0 0 0]  TranslationROffset=0  TranslationROffsetUnits=m  TranslationZOffset=0  TranslationZOffsetUnits=m  TranslationThetaOffset=0  TranslationThetaOffsetUnits=deg  RotationMethod=StandardAxis  RotationAngleUnits=deg  RotationStandardAxis=+Y  RotationAngle=90  RotationArbitraryAxis=[0 0 1]  FollAlignAxisA=+X  BaseAlignAxisA=+Y  FollAlignAxisB=+Y  BaseAlignAxisB=+Z  RotationSequenceAxes=FollowerAxes  RotationSequence=XYX  RotationSequenceAngles=[0 0 0]  RotationSequenceAnglesUnits=deg  RotationMatrix=[1 0 0; 0 1 0; 0 0 1]
  Rigid Transform2 : sm_lib/Frames and Transforms/Rigid Transform  TranslationMethod=Cartesian  TranslationStandardOffset=0  TranslationLengthUnit=m  TranslationStandardAxis=+Z  TranslationCartesianOffset=[-Rw 0 0]  TranslationROffset=0  TranslationROffsetUnits=m  TranslationZOffset=0  TranslationZOffsetUnits=m  TranslationThetaOffset=0  TranslationThetaOffsetUnits=deg  RotationMethod=None  RotationAngleUnits=deg  RotationStandardAxis=+Y  RotationAngle=90  RotationArbitraryAxis=[0 0 1]  FollAlignAxisA=+X  BaseAlignAxisA=+Y  FollAlignAxisB=+Y  BaseAlignAxisB=+Z  RotationSequenceAxes=FollowerAxes  RotationSequence=XYX  RotationSequenceAngles=[0 0 0]  RotationSequenceAnglesUnits=deg  RotationMatrix=[1 0 0; 0 1 0; 0 0 1]
  Rigid Transform3 : sm_lib/Frames and Transforms/Rigid Transform  TranslationMethod=Cartesian  TranslationStandardOffset=0  TranslationLengthUnit=m  TranslationStandardAxis=+Z  TranslationCartesianOffset=[0 0 0]  TranslationROffset=0  TranslationROffsetUnits=m  TranslationZOffset=0  TranslationZOffsetUnits=m  TranslationThetaOffset=0  TranslationThetaOffsetUnits=deg  RotationMethod=StandardAxis  RotationAngleUnits=deg  RotationStandardAxis=+X  RotationAngle=90  RotationArbitraryAxis=[0 0 1]  FollAlignAxisA=+X  BaseAlignAxisA=+Y  FollAlignAxisB=+Y  BaseAlignAxisB=+Z  RotationSequenceAxes=FollowerAxes  RotationSequence=XYX  RotationSequenceAngles=[0 0 0]  RotationSequenceAnglesUnits=deg  RotationMatrix=[1 0 0; 0 1 0; 0 0 1]
  Simulink-PS Converter{1..7} (7 alike) : nesl_utility/Simulink-PS Converter  PhysicalDomain=network_engine_domain  SubClassName=ps_input  LeftPortType=input  RightPortType=output  PseudoPeriodic=off  Frequencies=[]  NoiseDistribution=none  NoiseParameters=[]  Unit=1  AffineConversion=off  FilteringAndDerivatives=zero  SimscapeFilterOrder=1  InputFilterTimeConstant=0.001  UdotUserProvided=1
  Solver Configuration : nesl_utility/Solver Configuration  PhysicalDomain=network_engine_domain  SubClassName=solver  LeftPortType=input  RightPortType=generic  Tones=[]  Harmonics=[]  SimulateNoise=off  Profile=off  UseLocalSampling=off  EnableSwitchedLinearOptims=on  FrequencyDomain=off  UseCCode=off  RelTol=0.001  AbsTol=1e-06  MinStep=1e-09  ToWorkspace=off  RevertToSquareIcSolve=off  NumHomotopyIterations=100  PhasorMode=off  PhasorModeNumHarmonics=1  DoDC=off  ResidualTolerance=1e-09  UseLocalSolver=off  LocalSolverChoice=NE_BACKWARD_EULER_ADVANCER  LocalSolverSampleTime=0.001  DoFixedCost=off  MaxNonlinIter=3  MaxModeIter=2  LinearAlgebra=Sparse  EquationFormulation=NE_TIME_EF  DelaysMemoryBudget=1024  AutomaticFiltering=on  FilteringTimeConstant=0.001  PartitionStorageMethod=AS_NEEDED  PartitionMemoryBudget=1024  PartitionMethod=FAST
  Tiles : Subsystem
  Transform Rack3 : sm_lib/Frames and Transforms/Rigid Transform  TranslationMethod=StandardAxis  TranslationStandardOffset=0  TranslationLengthUnit=m  TranslationStandardAxis=-Z  TranslationCartesianOffset=[0 0 0]  TranslationROffset=0  TranslationROffsetUnits=m  TranslationZOffset=0  TranslationZOffsetUnits=m  TranslationThetaOffset=0  TranslationThetaOffsetUnits=deg  RotationMethod=None  RotationAngleUnits=deg  RotationStandardAxis=-X  RotationAngle=90  RotationArbitraryAxis=[0 0 1]  FollAlignAxisA=+X  BaseAlignAxisA=+Y  FollAlignAxisB=+Y  BaseAlignAxisB=+Z  RotationSequenceAxes=FollowerAxes  RotationSequence=XYX  RotationSequenceAngles=[0 0 0]  RotationSequenceAnglesUnits=deg  RotationMatrix=[1 0 0; 0 1 0; 0 0 1]
  World Frame : sm_lib/Frames and Transforms/World Frame
  wheelbot state : Selector  InputPortWidth=14  IndexOptions=Index vector (dialog)  Indices=[1 3 7 9 11 12 5]  OutputSizes=1
  wires:
  state/1 -> wheelbot state/1
  wheelbot state/1 -> Demux1/1
  Delay6/1 -> Simulink-PS Converter7/1
  Delay5/1 -> Simulink-PS Converter5/1
  Delay4/1 -> Simulink-PS Converter2/1
  Delay3/1 -> Simulink-PS Converter6/1
  Gain1/1 -> Delay3/1
  Delay2/1 -> Simulink-PS Converter4/1
  Delay1/1 -> Simulink-PS Converter1/1
  Delay/1 -> Simulink-PS Converter3/1
  Demux1/4 -> Gain3/1
  Demux1/3 -> Gain/1
  Gain3/1 -> Delay6/1
  Demux1/1 -> Delay2/1
  Demux1/6 -> Delay1/1
  Gain/1 -> Delay5/1
  Demux1/5 -> Delay/1
  Demux1/7 -> Delay4/1
  Demux1/2 -> Gain1/1
  connections:
  Rigid Transform3/LConn1 -- Rigid Transform2/RConn1
  Simulink-PS Converter2/RConn1 -- Planar Joint/LConn4
  Revolute Joint/LConn2 -- Simulink-PS Converter4/RConn1
  Chasis translation2/RConn1 -- Chasis translation3/LConn1
  Chasis translation3/RConn1 -- Revolute Joint3/LConn1
  Simulink-PS Converter1/RConn1 -- Planar Joint/LConn3
  Marker Wheel/LConn1 -- Revolute Joint1/RConn1 -- Ground-wheel/RConn1
  Chasis translation/LConn1 -- Revolute Joint2/RConn1
  Revolute Joint1/LConn2 -- Simulink-PS Converter5/RConn1
  Ground Plane/RConn1 -- Tiles/LConn1 -- Transform Rack3/RConn1
  Simulink-PS Converter3/RConn1 -- Planar Joint/LConn2
  Revolute Joint1/LConn1 -- Chasis translation1/LConn1 -- Rigid Transform3/RConn1
  Chasis translation1/RConn1 -- Revolute Joint2/LConn1
  Chasis/RConn1 -- Marker Chasis/LConn1 -- Chasis translation/RConn1 -- Chasis translation2/LConn1
  Revolute Joint3/LConn2 -- Simulink-PS Converter7/RConn1
  World Frame/RConn1 -- Planar Joint/LConn1 -- Solver Configuration/RConn1 -- Transform Rack3/LConn1
  Simulink-PS Converter6/RConn1 -- Revolute Joint2/LConn2
  Flywheel/RConn1 -- Revolute Joint3/RConn1 -- Marker Flywheel/LConn1
  Revolute Joint/LConn1 -- Rigid Transform1/RConn1
  Rigid Transform1/LConn1 -- Planar Joint/RConn1
  Rigid Transform2/LConn1 -- Revolute Joint/RConn1

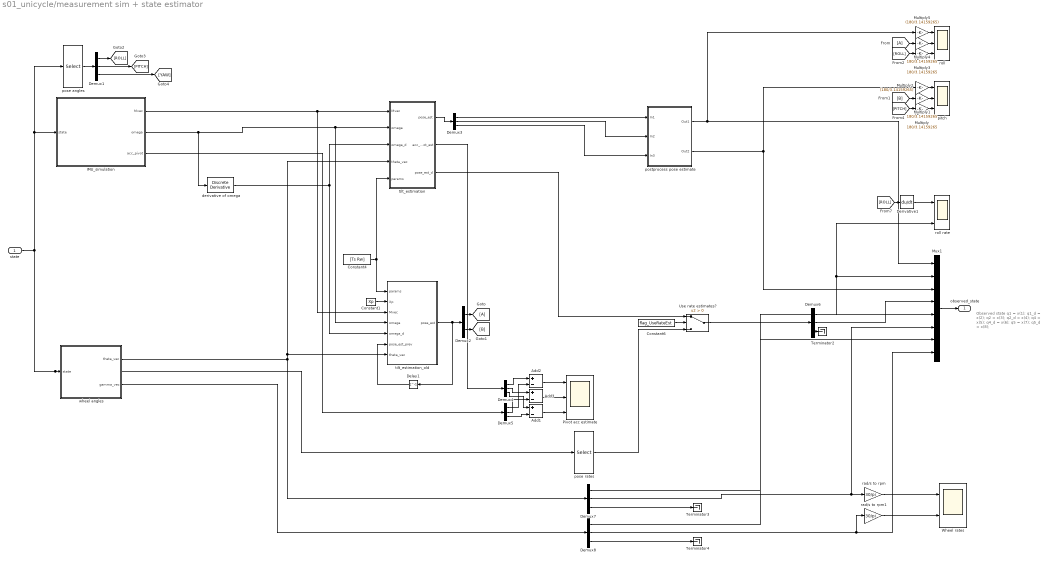
== system s01_unicycle/measurement sim + state estimator ==
  note: Observed state
      |
      | q1 = x(1);
      | q1_d = x(2);
      | q2 = x(3);
      | q2_d = x(4);
      | q4 = x(5);
      | q4_d = x(6);
      | q5 = x(7);
      | q5_d = x(8);
  state : Inport
  Add1 : Sum  Inputs=+-
  Add2 : Sum  Inputs=+-
  Add3 : Sum  Inputs=+-
  Constant1 : Constant  Value=Xp
  Constant4 : Constant  Value=[Ts Rw]
  Constant6 : Constant  Value=flag_UseRateEst
  Delay1 : Delay  DelayLength=1  InitialCondition=[q1_0; q2_0]  SampleTime=Ts
  Demux{1,3..8} (7 alike) : Demux  Outputs=3
  Demux2 : Demux  Outputs=2
  Derivative1 : Derivative
  IMU_simulation : Subsystem
      mask Display: image('IMU_block_image.PNG'); % Use "Edit Image" on toolstrip to change.
  Multiply{,1,3..4} (4 alike) : Gain  Gain=180/3.14159265
  Multiply2 : Gain  Gain=(180/3.14159265)
  Multiply5 : Gain  Gain=(180/3.14159265)
  Mux1 : Mux  Inputs=8
  Pivot acc estimate : Scope  NumInputPorts=3
  Terminator2 : Terminator
  Terminator3 : Terminator
  Terminator4 : Terminator
  Use rate estimates? : Switch  Criteria=u2 > Threshold
  Wheel rates : Scope  NumInputPorts=2
  derivative of omega : simulink/Discrete/Discrete Derivative  gainval=1.0  ICPrevScaledInput=0.0  OutMin=[]  OutMax=[]  OutDataType=fixdt(1, 16)  OutScaling=2^-10  DoSatur=off
  pitch : Scope  NumInputPorts=3
  pose angles : Selector  InputPortWidth=14  IndexOptions=Index vector (dialog)  Indices=[1,3, 5]  OutputSizes=1
  pose rates : Selector  InputPortWidth=14  IndexOptions=Index vector (dialog)  Indices=[2,4,6]  OutputSizes=1
  postprocess pose estimate : Subsystem
  rad/s to rpm : Gain  Gain=30/pi  SaturateOnIntegerOverflow=on  OutDataTypeStr=Inherit: Same as input  ParamDataTypeStr=Inherit: Same as input
  rad/s to rpm1 : Gain  Gain=30/pi  SaturateOnIntegerOverflow=on  OutDataTypeStr=Inherit: Same as input  ParamDataTypeStr=Inherit: Same as input
  roll : Scope  NumInputPorts=3
  roll rate : Scope  NumInputPorts=3
  tilt_estimation : Subsystem
  tilt_estimation_old : MATLAB Function  TreatAsAtomicUnit=on
  wheel angles : Subsystem
      mask Display: image('encoder_block_image.PNG'); % Use "Edit Image" on toolstrip to change.
  observed_state : Outport
  wires:
  IMU_simulation/2(omega) -> derivative of omega/1, tilt_estimation_old/4(omega), tilt_estimation/2(omega)
  IMU_simulation/1(Mvec) -> tilt_estimation_old/3(Mvec), tilt_estimation/1(Mvec)
  Constant4/1 -> tilt_estimation/5(params), tilt_estimation_old/1(params)
  tilt_estimation_old/1(pose_est) -> Delay1/1, Demux2/1
  Delay1/1 -> tilt_estimation_old/6(pose_est_prev)
  Demux4/1 -> Add2/1
  Demux5/1 -> Add2/2
  Add2/1 -> Pivot acc estimate/1
  Demux4/2 -> Add3/1
  Demux5/2 -> Add3/2
  Add3/1 -> Pivot acc estimate/2
  Multiply/1 -> pitch/3
  Multiply1/1 -> pitch/2
  Multiply2/1 -> pitch/1
  Multiply3/1 -> roll/3
  Multiply4/1 -> roll/2
  Multiply5/1 -> roll/1
  Demux3/2 -> postprocess pose estimate/2(In2)
  derivative of omega/1 -> tilt_estimation_old/5(omega_d), tilt_estimation/3(omega_d)
  tilt_estimation/2(acc_pivot_est) -> Demux4/1
  tilt_estimation/1(pose_est) -> Demux3/1
  IMU_simulation/3(acc_pivot) -> Demux5/1
  Constant1/1 -> tilt_estimation_old/2(Xp)
  state/1 -> pose rates/1, wheel angles/1(state), pose angles/1, IMU_simulation/1(state)
  pose angles/1 -> Demux1/1
  Demux2/1 -> [A]
  Demux2/2 -> [B]
  [A] -> Multiply4/1
  [B] -> Multiply1/1
  wheel angles/1(theta_vec) -> tilt_estimation/4(theta_vec), tilt_estimation_old/7(theta_vec), Demux7/1
  Mux1/1 -> observed_state/1
  Demux1/1 -> [ROLL]
  [ROLL] -> Multiply3/1
  Demux1/2 -> [PITCH]
  [PITCH] -> Multiply/1
  Demux4/3 -> Add1/1
  Demux5/3 -> Add1/2
  Add1/1 -> Pivot acc estimate/3
  Demux1/3 -> [YAW]
  pose rates/1 -> Use rate estimates?/3
  Demux6/1 -> roll rate/3, Mux1/2
  Demux6/2 -> Mux1/4
  Demux6/3 -> Terminator2/1
  tilt_estimation/3(pose_est_d) -> Use rate estimates?/1
  Use rate estimates?/1 -> Demux6/1
  Constant6/1 -> Use rate estimates?/2
  wheel angles/2(gamma_vec) -> Demux8/1
  Demux7/3 -> Terminator3/1
  Demux8/3 -> Terminator4/1
  Demux7/1 -> Mux1/5
  Demux7/2 -> rad/s to rpm/1, Mux1/6
  Demux8/1 -> Mux1/7
  Demux8/2 -> rad/s to rpm1/1, Mux1/8
  rad/s to rpm/1 -> Wheel rates/1
  rad/s to rpm1/1 -> Wheel rates/2
  Derivative1/1 -> roll rate/1
  [ROLL] -> Derivative1/1
  postprocess pose estimate/1(Out1) -> Mux1/1, Multiply5/1
  Demux3/1 -> postprocess pose estimate/1(In1)
  Demux3/3 -> postprocess pose estimate/3(In3)
  postprocess pose estimate/2(Out2) -> Mux1/3, Multiply2/1

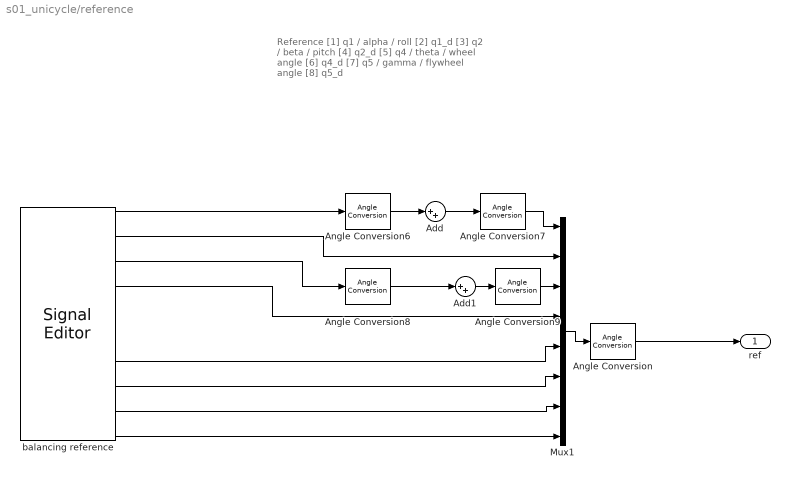
== system s01_unicycle/reference ==
  note: Reference
      |
      | [1] q1 / alpha / roll
      | [2] q1_d
      | [3] q2 / beta / pitch
      | [4] q2_d
      | [5] q4 / theta / wheel angle
      | [6] q4_d
      | [7] q5 / gamma / flywheel angle
      | [8] q5_d
  Add : Sum  Inputs=|++
  Add1 : Sum  Inputs=|++
  Angle Conversion : aerolibconvert2/Angle Conversion  IU=deg  OU=rad
  Angle Conversion6 : aerolibconvert2/Angle Conversion  IU=deg  OU=rad
  Angle Conversion7 : aerolibconvert2/Angle Conversion  IU=rad  OU=deg
  Angle Conversion8 : aerolibconvert2/Angle Conversion  IU=deg  OU=rad
  Angle Conversion9 : aerolibconvert2/Angle Conversion  IU=rad  OU=deg
  Mux1 : Mux  Inputs=8
  balancing reference : SignalEditorBlockLib/Signal Editor  FileName=C:\Users\geist\Documents\code_projects\uniwheel_model\simulink_3D_unicycle\signals\signal_reference.mat  ActiveScenario=q4d_and_q3d_slow_curve  ActiveSignal=q2  IsBus=off  OutputBusObjectStr=Bus: BusObject  SampleTime=0  ZeroCross=off  OutputAfterFinalValue=Setting to zero  Unit=inherit  PreserveSignalName=on
  ref : Outport
  wires:
  balancing reference/7 -> Mux1/5
  balancing reference/1 -> Angle Conversion6/1
  balancing reference/8 -> Mux1/6
  balancing reference/2 -> Mux1/2
  balancing reference/3 -> Angle Conversion8/1
  balancing reference/4 -> Mux1/4
  balancing reference/9 -> Mux1/7
  balancing reference/10 -> Mux1/8
  Mux1/1 -> Angle Conversion/1
  Angle Conversion/1 -> ref/1
  Add/1 -> Angle Conversion7/1
  Angle Conversion6/1 -> Add/1
  Angle Conversion7/1 -> Mux1/1
  Angle Conversion8/1 -> Add1/1
  Angle Conversion9/1 -> Mux1/3
  Add1/1 -> Angle Conversion9/1

== system s01_unicycle/animation/Marker Chasis ==
  String7 (Graphic) : sm_lib/Body Elements/Brick Solid  GraphicAmbientColor=[0.15 0.15 0.15 1.0]  BasedOnType=Density  BrickDimensions=[0.003 Lcp+Lc+0.01 0.045]  BrickDimensionUnits=m  CenterOfMass=[0 0 0]  CenterOfMassUnits=m  GraphicDiffuseColor=[0.0 0.0 0.0]  Density=0  DensityUnits=kg/(m^3)  DoExposeReferenceFrame=on  GraphicEmissiveColor=[0.0 0.0 0.0 1.0]  ExportEntireGeometry=off  SerializedFrames=<Frames/>  MarkerShape=Sphere  MarkerSize=10  GraphicType=FromGeometry  InertiaType=PointMass  Mass=0  MassUnits=kg  MomentsOfInertia=[1 1 1]*1e-3  MomentsOfInertiaUnits=kg*m^2  GraphicOpacity=1.0  ProductsOfInertia=[0 0 0]  ProductsOfInertiaUnits=kg*m^2  GraphicShininess=75  GraphicSpecularColor=[0.5 0.5 0.5 1.0]  GraphicVisPropType=SimpleVisualProperties
  String8 (Graphic) : sm_lib/Body Elements/Brick Solid  GraphicAmbientColor=[0.15 0.15 0.15 1.0]  BasedOnType=Density  BrickDimensions=[0.003 0.045 0.045]  BrickDimensionUnits=m  CenterOfMass=[0 0 0]  CenterOfMassUnits=m  GraphicDiffuseColor=[0.0 0.0 0.0]  Density=0  DensityUnits=kg/(m^3)  DoExposeReferenceFrame=on  GraphicEmissiveColor=[0.0 0.0 0.0 1.0]  ExportEntireGeometry=off  SerializedFrames=<Frames/>  MarkerShape=Sphere  MarkerSize=10  GraphicType=FromGeometry  InertiaType=PointMass  Mass=0  MassUnits=kg  MomentsOfInertia=[1 1 1]*1e-3  MomentsOfInertiaUnits=kg*m^2  GraphicOpacity=1.0  ProductsOfInertia=[0 0 0]  ProductsOfInertiaUnits=kg*m^2  GraphicShininess=75  GraphicSpecularColor=[0.5 0.5 0.5 1.0]  GraphicVisPropType=SimpleVisualProperties
  Transform String Midpoint14 : sm_lib/Frames and Transforms/Rigid Transform  TranslationMethod=None  TranslationStandardOffset=1  TranslationLengthUnit=m  TranslationStandardAxis=+Y  TranslationCartesianOffset=[0 0 0]  TranslationROffset=0  TranslationROffsetUnits=m  TranslationZOffset=0  TranslationZOffsetUnits=m  TranslationThetaOffset=0  TranslationThetaOffsetUnits=deg  RotationMethod=StandardAxis  RotationAngleUnits=deg  RotationStandardAxis=+Z  RotationAngle=90  RotationArbitraryAxis=[0 0 1]  FollAlignAxisA=+X  BaseAlignAxisA=+Y  FollAlignAxisB=+Y  BaseAlignAxisB=+Z  RotationSequenceAxes=FollowerAxes  RotationSequence=XYX  RotationSequenceAngles=[0 0 0]  RotationSequenceAnglesUnits=deg  RotationMatrix=[1 0 0; 0 1 0; 0 0 1]
  Conn1 : PMIOPort  Side=Left
  connections:
  String8 (Graphic)/RConn1 -- Transform String Midpoint14/RConn1
  String7 (Graphic)/RConn1 -- Conn1/RConn1 -- Transform String Midpoint14/LConn1

== system s01_unicycle/animation/Marker Flywheel ==
  String1 : sm_lib/Body Elements/Brick Solid  GraphicAmbientColor=[0.15 0.15 0.15 1.0]  BasedOnType=Density  BrickDimensions=[0.001 2*Rw b_disc]  BrickDimensionUnits=m  CenterOfMass=[0 0 0]  CenterOfMassUnits=m  GraphicDiffuseColor=[1 0 0]  Density=0  DensityUnits=kg/(m^3)  DoExposeReferenceFrame=on  GraphicEmissiveColor=[0.0 0.0 0.0 1.0]  ExportEntireGeometry=off  SerializedFrames=<Frames/>  MarkerShape=Sphere  MarkerSize=10  GraphicType=FromGeometry  InertiaType=PointMass  Mass=0  MassUnits=kg  MomentsOfInertia=[1 1 1]*1e-3  MomentsOfInertiaUnits=kg*m^2  GraphicOpacity=1.0  ProductsOfInertia=[0 0 0]  ProductsOfInertiaUnits=kg*m^2  GraphicShininess=75  GraphicSpecularColor=[0.5 0.5 0.5 1.0]  GraphicVisPropType=SimpleVisualProperties
  String2 : sm_lib/Body Elements/Brick Solid  GraphicAmbientColor=[0.15 0.15 0.15 1.0]  BasedOnType=Density  BrickDimensions=[0.001 2*Rw b_disc]  BrickDimensionUnits=m  CenterOfMass=[0 0 0]  CenterOfMassUnits=m  GraphicDiffuseColor=[1 0 0]  Density=0  DensityUnits=kg/(m^3)  DoExposeReferenceFrame=on  GraphicEmissiveColor=[0.0 0.0 0.0 1.0]  ExportEntireGeometry=off  SerializedFrames=<Frames/>  MarkerShape=Sphere  MarkerSize=10  GraphicType=FromGeometry  InertiaType=PointMass  Mass=0  MassUnits=kg  MomentsOfInertia=[1 1 1]*1e-3  MomentsOfInertiaUnits=kg*m^2  GraphicOpacity=1.0  ProductsOfInertia=[0 0 0]  ProductsOfInertiaUnits=kg*m^2  GraphicShininess=75  GraphicSpecularColor=[0.5 0.5 0.5 1.0]  GraphicVisPropType=SimpleVisualProperties
  Transform String Midpoint1 : sm_lib/Frames and Transforms/Rigid Transform  TranslationMethod=None  TranslationStandardOffset=1  TranslationLengthUnit=m  TranslationStandardAxis=+Y  TranslationCartesianOffset=[0 0 0]  TranslationROffset=0  TranslationROffsetUnits=m  TranslationZOffset=0  TranslationZOffsetUnits=m  TranslationThetaOffset=0  TranslationThetaOffsetUnits=deg  RotationMethod=StandardAxis  RotationAngleUnits=deg  RotationStandardAxis=+Z  RotationAngle=90  RotationArbitraryAxis=[0 0 1]  FollAlignAxisA=+X  BaseAlignAxisA=+Y  FollAlignAxisB=+Y  BaseAlignAxisB=+Z  RotationSequenceAxes=FollowerAxes  RotationSequence=XYX  RotationSequenceAngles=[0 0 0]  RotationSequenceAnglesUnits=deg  RotationMatrix=[1 0 0; 0 1 0; 0 0 1]
  Conn1 : PMIOPort  Side=Left
  connections:
  String2/RConn1 -- Transform String Midpoint1/RConn1
  Transform String Midpoint1/LConn1 -- Conn1/RConn1 -- String1/RConn1

== system s01_unicycle/animation/Marker Wheel ==
  String11 : sm_lib/Body Elements/Brick Solid  GraphicAmbientColor=[0.15 0.15 0.15 1.0]  BasedOnType=Density  BrickDimensions=[0.001 2*Rw b_disc]  BrickDimensionUnits=m  CenterOfMass=[0 0 0]  CenterOfMassUnits=m  GraphicDiffuseColor=[0 0.0 1.0]  Density=0  DensityUnits=kg/(m^3)  DoExposeReferenceFrame=on  GraphicEmissiveColor=[0.0 0.0 0.0 1.0]  ExportEntireGeometry=off  SerializedFrames=<Frames/>  MarkerShape=Sphere  MarkerSize=10  GraphicType=FromGeometry  InertiaType=PointMass  Mass=0  MassUnits=kg  MomentsOfInertia=[1 1 1]*1e-3  MomentsOfInertiaUnits=kg*m^2  GraphicOpacity=1.0  ProductsOfInertia=[0 0 0]  ProductsOfInertiaUnits=kg*m^2  GraphicShininess=75  GraphicSpecularColor=[0.5 0.5 0.5 1.0]  GraphicVisPropType=SimpleVisualProperties
  String12 : sm_lib/Body Elements/Brick Solid  GraphicAmbientColor=[0.15 0.15 0.15 1.0]  BasedOnType=Density  BrickDimensions=[0.001 2*Rw b_disc]  BrickDimensionUnits=m  CenterOfMass=[0 0 0]  CenterOfMassUnits=m  GraphicDiffuseColor=[0 0 1]  Density=0  DensityUnits=kg/(m^3)  DoExposeReferenceFrame=on  GraphicEmissiveColor=[0.0 0.0 0.0 1.0]  ExportEntireGeometry=off  SerializedFrames=<Frames/>  MarkerShape=Sphere  MarkerSize=10  GraphicType=FromGeometry  InertiaType=PointMass  Mass=0  MassUnits=kg  MomentsOfInertia=[1 1 1]*1e-3  MomentsOfInertiaUnits=kg*m^2  GraphicOpacity=1.0  ProductsOfInertia=[0 0 0]  ProductsOfInertiaUnits=kg*m^2  GraphicShininess=75  GraphicSpecularColor=[0.5 0.5 0.5 1.0]  GraphicVisPropType=SimpleVisualProperties
  Transform String Midpoint12 : sm_lib/Frames and Transforms/Rigid Transform  TranslationMethod=None  TranslationStandardOffset=1  TranslationLengthUnit=m  TranslationStandardAxis=+Y  TranslationCartesianOffset=[0 0 0]  TranslationROffset=0  TranslationROffsetUnits=m  TranslationZOffset=0  TranslationZOffsetUnits=m  TranslationThetaOffset=0  TranslationThetaOffsetUnits=deg  RotationMethod=StandardAxis  RotationAngleUnits=deg  RotationStandardAxis=+Z  RotationAngle=90  RotationArbitraryAxis=[0 0 1]  FollAlignAxisA=+X  BaseAlignAxisA=+Y  FollAlignAxisB=+Y  BaseAlignAxisB=+Z  RotationSequenceAxes=FollowerAxes  RotationSequence=XYX  RotationSequenceAngles=[0 0 0]  RotationSequenceAnglesUnits=deg  RotationMatrix=[1 0 0; 0 1 0; 0 0 1]
  Conn1 : PMIOPort  Side=Left
  connections:
  String12/RConn1 -- Transform String Midpoint12/RConn1
  String11/RConn1 -- Conn1/RConn1 -- Transform String Midpoint12/LConn1
